simulink model "F16_trim"  (Simulink 6.0)
settings: Solver=ode45  StartTime=0.0  StopTime=10.0  RelTol=1e-3
settings Model: Creator=larssonneveldt  LastModifiedBy=larssonneveldt
settings DataIOCC: SignalLoggingName=sigsOut
settings DebuggingCC: SolverPrmCheckMsg=none  MultiTaskDSMMsg=warning  MultiTaskCondExecSysMsg=none  FcnCallInpInsideContextMsg=Use local settings  StrictBusMsg=None
settings HardwareCC: TargetHWDeviceType=32-bit Generic  TargetUnknown=on  ProdEqTarget=off
settings RTWCC: IncludeERTFirstTime=on
settings CodeAppCC: CustomSymbolStrType=$N$R$M

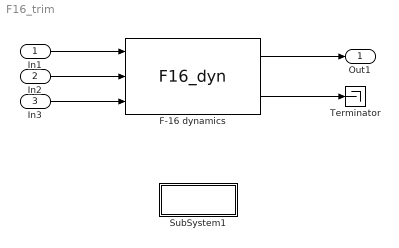
== system F16_trim ==
  In1 : Inport  OutDataType=sfix(16)  OutScaling=2^0
  In2 : Inport  Port=2  OutDataType=sfix(16)  OutScaling=2^0
  In3 : Inport  Port=3  OutDataType=sfix(16)  OutScaling=2^0
  F-16 dynamics : S-Function  FunctionName=F16_dyn  Parameters="[100 0 14.74*pi/180, cos(14.74*pi/360) 0 sin(14.74*pi/360)  0, 0 0 0, 0 0 -5000 20]"  EnableBusSupport=off
      mask Display: image(imread('aerodata/f16.jpg'))
  SubSystem1 : Subsystem
      settings: OpenFcn=edit(fullfile(cd,'F16_dyn.c'))
      mask Display: disp('F16_dyn.c');
  Terminator : Terminator
  Out1 : Outport  OutDataType=sfix(16)  OutScaling=2^0
  wires:
  F-16 dynamics/1 -> Out1/1
  In3/1 -> F-16 dynamics/3
  In1/1 -> F-16 dynamics/1
  In2/1 -> F-16 dynamics/2
  F-16 dynamics/2 -> Terminator/1

== system F16_trim/SubSystem1 ==
